simulink model "controlBiomasaAP"  (R2018a)
settings: Solver=FixedStepAuto  StartTime=0.0  StopTime=10000  RelTol=1e-3
values from neighbouring files (symbols this model uses):
  A = [S.A zeros(n,p); -S.C eye(p)]    [poles_int.m]
  c = cr(i)    [MetodosNumericos.m]
  ce = zeros(1,n)    [MetodosNumericos.m]
  q0 = eval(solucionParam.qs0)    [discretizacion.m]
  q1 = eval(solucionParam.qs1)    [discretizacion.m]
  q2 = eval(solucionParam.qs2)    [discretizacion.m]
  r1 = eval(solucionParam.rs1)    [discretizacion.m]
undefined symbols (not defined in the file or in its folder): BM, C, D, x
libraries: simulink x3
settings Model: Creator=Asus  LastModifiedBy=mvasqu49
settings CodeAppCC: StateflowObjectComments=on

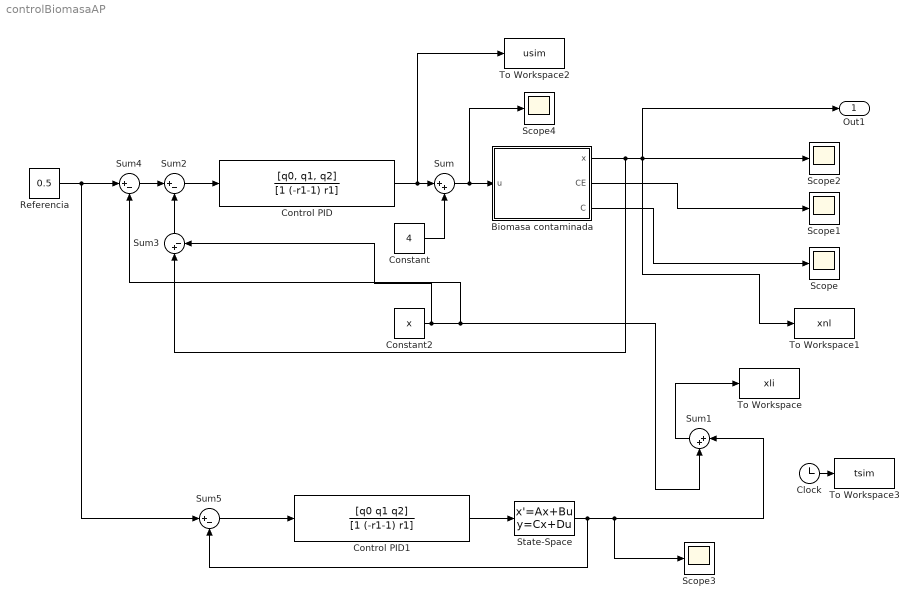
== system controlBiomasaAP ==
  Biomasa contaminada : Subsystem  mask(Modelo){par=[0.01, 0.01,0.2,0.2,0.1,0.1,5,0.01,2], ci=[x,c,ce]}
      mask prompts: par "[n, a, b, h, mu, r0, k0, r1, p]"; ci "[x0, c0, ce0]"
      mask help:
      | Modelo de concentración de contaminación en un ambiente
      | Entrada: contaminación
      | Salidas: biomasa de la población (x), concentración de toxina en el ambiente (Ce), cantidad de toxina en la biomasa de la población (C)
      mask init:
      | n  = par(1);
      | a  = par(2); 
      | b  = par(3);
      | h  = par(4);
      | mu = par(5); 
      | r0 = par(6); 
      | k0 = par(7); 
      | r1 = par(8); 
      | p  = par(9); 
      | x0 = ci(1);
      | c0 = ci(2);
      | ce0 = ci(3);
  Clock : Clock
  Constant : Constant  Value=4  SampleTime=0.5
  Constant2 : Constant  Value=x
  Control PID : DiscreteTransferFcn  Numerator=[q0, q1, q2]  Denominator=[1 (-r1-1) r1]  SampleTime=0.5
  Control PID1 : DiscreteTransferFcn  Numerator=[q0 q1 q2]  Denominator=[1 (-r1-1) r1]  SampleTime=0.5
  Referencia : Constant  Value=0.5  SampleTime=0.5
  Scope{,1..4} (5 alike) : Scope
  State-Space : StateSpace  A=A  B=BM  C=C  D=D  InitialCondition=0
  Sum : Sum  Inputs=|++
  Sum1 : Sum  Inputs=|++
  Sum{2..5} (4 alike) : Sum  Inputs=|+-
  To Workspace : ToWorkspace  VariableName=xli  SampleTime=-1
  To Workspace1 : ToWorkspace  VariableName=xnl  SampleTime=-1
  To Workspace2 : ToWorkspace  VariableName=usim  SampleTime=-1
  To Workspace3 : ToWorkspace  VariableName=tsim  SampleTime=-1
  Out1 : Outport
  wires:
  Biomasa contaminada/1(x) -> Sum3/1, Scope2/1, Out1/1, To Workspace1/1
  Biomasa contaminada/2(CE) -> Scope1/1
  Biomasa contaminada/3(C) -> Scope/1
  State-Space/1 -> Sum5/2, Scope3/1, Sum1/1
  Sum1/1 -> To Workspace/1
  Constant2/1 -> Sum3/2, Sum4/2, Sum1/2
  Clock/1 -> To Workspace3/1
  Sum2/1 -> Control PID/1
  Constant/1 -> Sum/2
  Sum/1 -> Scope4/1, Biomasa contaminada/1(u)
  Sum3/1 -> Sum2/2
  Control PID/1 -> To Workspace2/1, Sum/1
  Control PID1/1 -> State-Space/1
  Referencia/1 -> Sum5/1, Sum4/1
  Sum4/1 -> Sum2/1
  Sum5/1 -> Control PID1/1

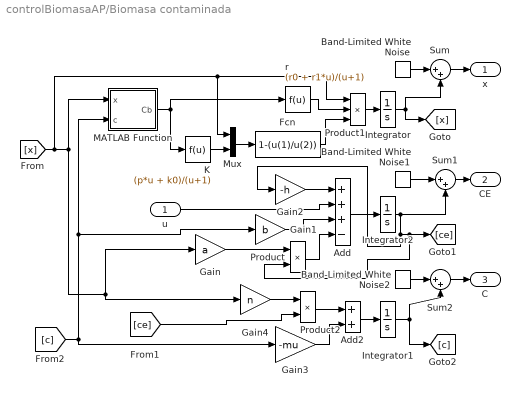
== system controlBiomasaAP/Biomasa contaminada ==
  u : Inport
  Add : Sum  Inputs=+++-
  Add2 : Sum
  Band-Limited White Noise : simulink/Sources/Band-Limited White Noise  Cov=0  Ts=0.1  seed=[1542869]
  Band-Limited White Noise1 : simulink/Sources/Band-Limited White Noise  Cov=0  Ts=0.1  seed=[4785963]
  Band-Limited White Noise2 : simulink/Sources/Band-Limited White Noise  Cov=0  Ts=0.1  seed=[5468953]
  Fcn : Fcn  Expr=1-(u(1)/u(2))
  Gain : Gain  Gain=a
  Gain1 : Gain  Gain=b
  Gain2 : Gain  Gain=-h
  Gain3 : Gain  Gain=-mu
  Gain4 : Gain  Gain=n
  Integrator : Integrator  InitialCondition=x0
  Integrator1 : Integrator  InitialCondition=c0
  Integrator2 : Integrator  InitialCondition=ce0
  "K " : Fcn  Expr=(p*u + k0)/(u+1)
  MATLAB Function : MATLAB Function  TreatAsAtomicUnit=on
  Mux : Mux  Inputs=2
  Product : Product
  Product1 : Product  Inputs=3
  Product2 : Product
  Sum : Sum  Inputs=|++
  Sum1 : Sum  Inputs=|++
  Sum2 : Sum  Inputs=|++
  "r " : Fcn  Expr=(r0 + r1*u)/(u+1)
  x : Outport
  CE : Outport  Port=2
  C : Outport  Port=3
  wires:
  Product/1 -> Add/4
  Gain1/1 -> Add/3
  Product1/1 -> Integrator/1
  Mux/1 -> Fcn/1
  u/1 -> Add/2
  Gain2/1 -> Add/1
  Add/1 -> Integrator2/1
  MATLAB Function/1(Cb) -> "r "/1, "K "/1
  "r "/1 -> Product1/2
  Integrator/1 -> Sum/2, [x]
  Fcn/1 -> Product1/3
  [x] -> Mux/1, Product1/1, MATLAB Function/1(x), Gain4/1, Gain/1
  [c] -> Gain1/1, MATLAB Function/2(c), Gain3/1
  [ce] -> Product2/2
  Gain4/1 -> Product2/1
  Product2/1 -> Add2/1
  Gain3/1 -> Add2/2
  Add2/1 -> Integrator1/1
  Integrator1/1 -> Sum2/2, [c]
  Gain/1 -> Product/1
  "K "/1 -> Mux/2
  Sum/1 -> x/1
  Band-Limited White Noise/1 -> Sum/1
  Band-Limited White Noise1/1 -> Sum1/1
  Sum1/1 -> CE/1
  Integrator2/1 -> Product/2, [ce], Gain2/1, Sum1/2
  Band-Limited White Noise2/1 -> Sum2/1
  Sum2/1 -> C/1

== matlab function controlBiomasaAP/Biomasa contaminada/MATLAB Function ==
  data: x input; c input; Cb output
function Cb = fcn(x, c)
if x == 0
    Cb = 0;
else
    Cb = c/x;
end
end
